simulink model "Colorspace_Conv_Plus_Padding"  (Simulink 6.4)
settings: Solver=ode45  StartTime=0.0  StopTime=5  RelTol=1e-3
undefined symbols (not defined in the file): jet, Rec, SDTV
libraries: vipconversions x4, vipsnks x2, viputilities x1, vipsrcs x1
settings Model: LastModifiedBy=Pr . Saddam&Ali

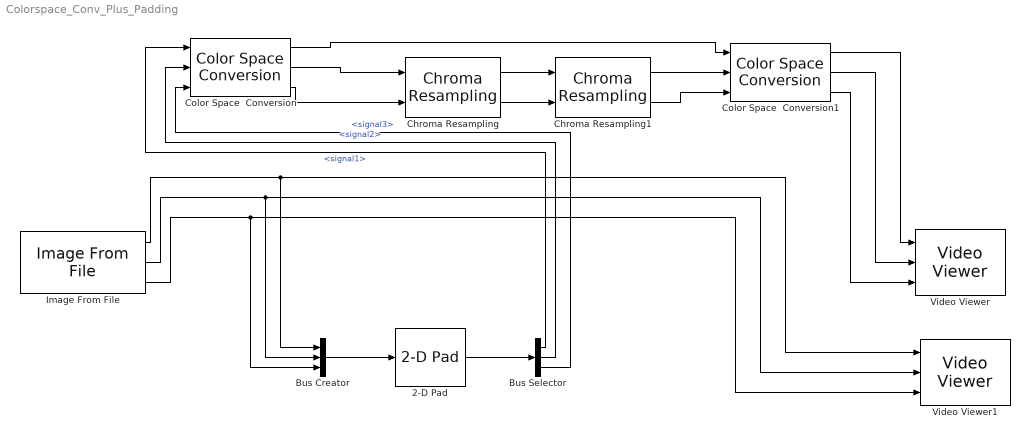
== system Colorspace_Conv_Plus_Padding ==
  2-D Pad : viputilities/2-D Pad  method=Replicate  valSrc=Specify via dialog  value=0  spec=Pad size  rowDirection=Right  rowSize=1  outColSize=10  colDirection=Both top and bottom  colSize=[2 3]  outRowSize=12
  Bus Creator : BusCreator  Inputs=3
  Bus Selector : BusSelector  OutputSignals=signal1,signal2,signal3
  Chroma Resampling : vipconversions/Chroma Resampling  resampling=4:4:4 to 4:2:2  interpolation=linear  antialiasing=Default  hcoeff=[0.2 0.6 0.2]  vcoeff=[0.5 0.5]
  Chroma Resampling1 : vipconversions/Chroma Resampling  resampling=4:2:2 to 4:4:4  interpolation=linear  antialiasing=Default  hcoeff=[0.2 0.6 0.2]  vcoeff=[0.5 0.5]
  Color Space  Conversion : vipconversions/Color Space  Conversion  conversion=R'G'B' to Y'CbCr  wp_str=D65  rec=Rec. 601 (SDTV)  sys=1125/60/2:1
  Color Space  Conversion1 : vipconversions/Color Space  Conversion  conversion=Y'CbCr to R'G'B'  wp_str=D65  rec=Rec. 601 (SDTV)  sys=1125/60/2:1
  Image From File : vipsrcs/Image From File  DialogController=vipDDGCreate  DialogControllerArgs=DataTag0  SystemSampleTime=-1  FileName=D:\A l i\FCI_4th Year\2nd Term\Void\ID 2.JPG  Ts=inf  ImageDataType=Inherit from input image  Signed=on  WordLength=16  sdImageDataType=uint(8)  FractionLengthMode=User-defined  FractionLength=15  OutPortLabels=R|G|B
  Video Viewer : vipsnks/Video Viewer  inputType=RGB  useColorMap=off  colormapValue=jet(256);  specRange=off  minInputVal=0  maxInputVal=255  FigPos=[256 264 512 384]  AxisZoom=on  trueSizedOnce=on
  Video Viewer1 : vipsnks/Video Viewer  inputType=RGB  useColorMap=off  colormapValue=jet(256);  specRange=off  minInputVal=0  maxInputVal=255  FigPos=[256 264 512 384]  AxisZoom=on  trueSizedOnce=on
  wires:
  Color Space  Conversion/1 -> Color Space  Conversion1/1
  Image From File/1 -> Video Viewer1/1, Bus Creator/1
  Image From File/2 -> Video Viewer1/2, Bus Creator/2
  Image From File/3 -> Video Viewer1/3, Bus Creator/3
  Color Space  Conversion/2 -> Chroma Resampling/1
  Color Space  Conversion/3 -> Chroma Resampling/2
  Chroma Resampling/1 -> Chroma Resampling1/1
  Chroma Resampling/2 -> Chroma Resampling1/2
  Chroma Resampling1/1 -> Color Space  Conversion1/2
  Chroma Resampling1/2 -> Color Space  Conversion1/3
  Color Space  Conversion1/1 -> Video Viewer/1
  Color Space  Conversion1/2 -> Video Viewer/2
  Color Space  Conversion1/3 -> Video Viewer/3
  Bus Creator/1 -> 2-D Pad/1
  2-D Pad/1 -> Bus Selector/1
  Bus Selector/1 -> Color Space  Conversion/1  "<signal1>"
  Bus Selector/2 -> Color Space  Conversion/2  "<signal2>"
  Bus Selector/3 -> Color Space  Conversion/3  "<signal3>"
